simulink model "project2"  (R2023a)
settings: Solver=ode23tb  StartTime=0.0  StopTime=10.0  MaxStep=1e-3  RelTol=1e-3
InitFcn:
  | Ra=0.6;
  | La=12e-3;
  | Rf=240;
  | Lf=120;
  | j=1;
  | K=1.309;
libraries: spsDiodeLib x8, spsSeriesRLCBranchLib x6, spsMeanLib x4, slpidlib x4, spsControlledVoltageSourceLib x4, spsCurrentMeasurementLib x4, simulink x3, spsACVoltageSourceLib x2, spsDCVoltageSourceLib x2, spsVoltageMeasurementLib x2, sps_lib x1
settings Model: Creator=gaming3  LastModifiedBy=gaming3
settings SolverCC: ZeroCrossAlgorithm=Adaptive
settings DebuggingCC: IgnoredZcDiagnostic=none

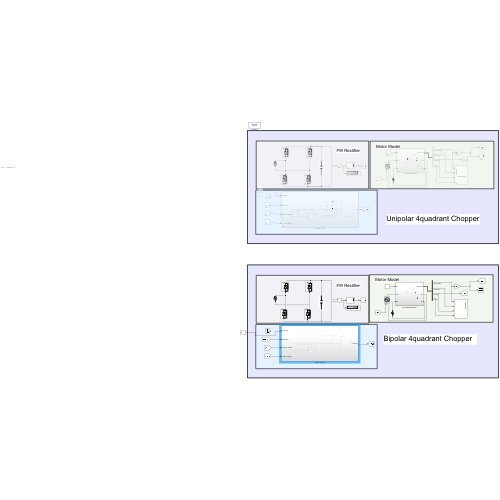
[thumbnail: Simulink's stored preview of the top-level diagram]
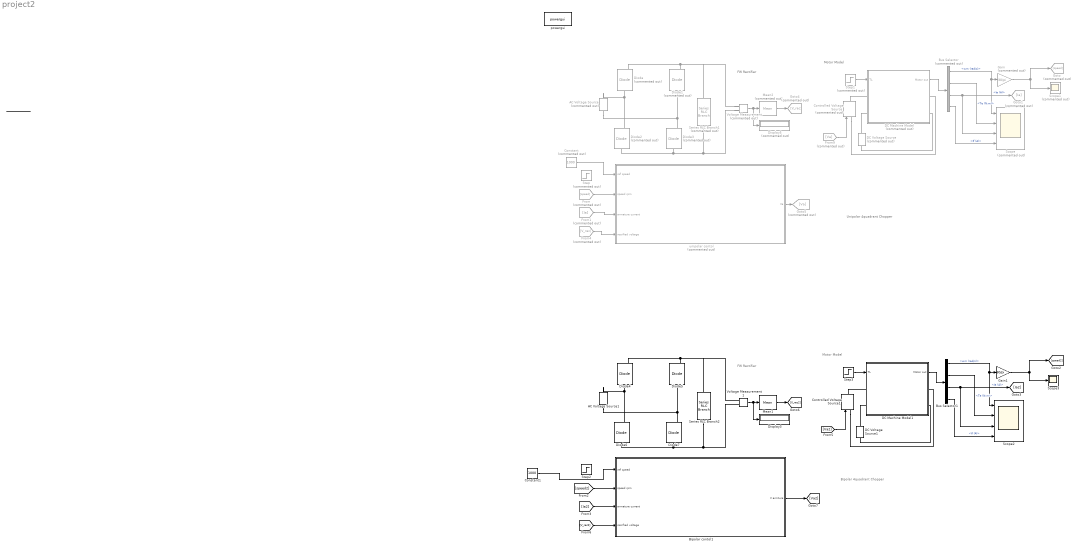
== system project2 ==
  note: Unipolar 4quadrant Chopper
  note: FW Rectifier
  note: Motor Model
  note: Bipolar 4quadrant Chopper
  note: FW Rectifier
  note: Motor Model
  AC Voltage Source : spsACVoltageSourceLib/AC Voltage Source  Commented=on  Amplitude=220  Phase=0  Frequency=50  SampleTime=0  Measurements=None  BusType=swing  Pref=10e3  Qref=0  Qmin=-inf  Qmax=+inf
  AC Voltage Source1 : spsACVoltageSourceLib/AC Voltage Source  Amplitude=220  Phase=0  Frequency=50  SampleTime=0  Measurements=None  BusType=swing  Pref=10e3  Qref=0  Qmin=-inf  Qmax=+inf
  Bipolar contol1 : Subsystem
  Bus Selector : BusSelector  Commented=on  OutputSignals=wm (rad/s),Te (N:m),Ia (A),If (A)
  Bus Selector1 : BusSelector  OutputSignals=wm (rad/s),Te (N:m),Ia (A),If (A)
  Constant : Constant  Commented=on  Value=1000
  Constant1 : Constant  Value=1000
  Controlled Voltage Source : spsControlledVoltageSourceLib/Controlled Voltage Source  Commented=on  Initialize=on  Source_Type=DC  Amplitude=0  Phase=0  Frequency=0  Measurements=None
  Controlled Voltage Source1 : spsControlledVoltageSourceLib/Controlled Voltage Source  Initialize=on  Source_Type=DC  Amplitude=0  Phase=0  Frequency=0  Measurements=None
  DC Machine Model : Subsystem  Commented=on
  DC Machine Model1 : Subsystem
  DC Voltage Source : spsDCVoltageSourceLib/DC Voltage Source  Commented=on  Amplitude=300  Measurements=None
  DC Voltage Source1 : spsDCVoltageSourceLib/DC Voltage Source  Amplitude=300  Measurements=None
  Diode{,1..3} (4 alike) : spsDiodeLib/Diode  Commented=on  Ron=0.001  Lon=0  Vf=0.8  IC=0  UseSnubber=0  Rs=500  Cs=250e-9  Measurements=on
  Diode{4..7} (4 alike) : spsDiodeLib/Diode  Ron=0.001  Lon=0  Vf=0.8  IC=0  UseSnubber=0  Rs=500  Cs=250e-9  Measurements=on
  Display3 : Display
  Display5 : Display  Commented=on
  From : From  Commented=on  GotoTag=speed
  From1 : From  Commented=on  GotoTag=Ia
  From4 : From  Commented=on  GotoTag=V_rec
  From9 : From  Commented=on  GotoTag=Va
  Gain : Gain  Commented=on  Gain=30/pi
  Gain1 : Gain  Gain=30/pi
  Goto : Goto  Commented=on  GotoTag=speed
  Goto1 : Goto  Commented=on  GotoTag=Ia
  Goto4 : Goto  Commented=on  GotoTag=V_rec
  Goto5 : Goto  Commented=on  GotoTag=Va
  Mean1 : spsMeanLib/Mean  Freq=50  Vinit=0  Ts=0
  Mean2 : spsMeanLib/Mean  Commented=on  Freq=50  Vinit=0  Ts=0
  Scope : Scope  Commented=on  NumInputPorts=4
  Scope1 : Scope  Commented=on
  Scope2 : Scope  NumInputPorts=4
  Scope3 : Scope
  Series RLC Branch1 : spsSeriesRLCBranchLib/Series RLC Branch  Commented=on  LConnTagsString=__new0  RConnTagsString=__new0  BranchType=C  Resistance=1  Inductance=1e-3  SetiL0=off  InitialCurrent=0  Capacitance=2  Setx0=off  InitialVoltage=0  Measurements=None
  Series RLC Branch2 : spsSeriesRLCBranchLib/Series RLC Branch  LConnTagsString=__new0  RConnTagsString=__new0  BranchType=C  Resistance=1  Inductance=1e-3  SetiL0=off  InitialCurrent=0  Capacitance=2  Setx0=off  InitialVoltage=0  Measurements=None
  Step : Step  Commented=on  Time=5  Before=700  After=-700  SampleTime=0
  Step1 : Step  Commented=on  Time=5  Before=70  After=100  SampleTime=0
  Step2 : Step  Time=5  Before=700  After=-700  SampleTime=0
  Step3 : Step  Time=5  Before=20  After=60  SampleTime=0
  Voltage Measurement : spsVoltageMeasurementLib/Voltage Measurement  Commented=on  PhasorSimulation=off  OutputType=Complex  PSBequivalent=0
  Voltage Measurement1 : spsVoltageMeasurementLib/Voltage Measurement  PhasorSimulation=off  OutputType=Complex  PSBequivalent=0
  powergui : sps_lib/powergui  Priority=1  SimulationMode=Discrete  SampleTime=10e-6  frequency=60  Iterations=50  frequencyindice=0  Pbase=100e6  ErrMax=1e-4  UnitsV=kV  UnitsW=MW  buscounter=0  FunctionMessages=off  echomessages=off  EnableUseOfTLC=off  CurrentSourceSwitches=off  DisableSnubberDevices=off  DisableRonSwitches=off  DisableVfSwitches=off  DisplayEquations=off  AutomaticDiscreteSolvers=off  SolverType=Tustin/Backward Euler (TBE)  Interpol=off  ExternalGateDelay=off  methode=off  Ts=100  x0status=blocks  SPID=on  SwTol=0  HookPort=off  NonlinearTolerance=1e-4  nMaxIteration=100  ContinueOnMaxIteration=off  RestoreLinks=warning  ResistiveCurrentMeasurement=off  Frange=[0:2:500]  Ylog=off  Xlog=on  ShowGrid=off  save=off  variable=ZData  structure=0  ZoomFFT=off  StartTime=0.0  cycles=1  DisplayStyle=1  fundamental=60  FreqAxis=off  MaxFrequency=1000  frequencyindicesteady=1  RmsSteady=1  display=off
  unipolar contol : Subsystem  Commented=on
  wires:
  Gain/1 -> Scope1/1, Goto/1
  Voltage Measurement/1 -> Mean2/1, Display5/1
  From/1 -> unipolar contol/2(speed rpm)
  From1/1 -> unipolar contol/3(armature current)
  Mean2/1 -> Goto4/1
  From4/1 -> unipolar contol/4(recrified voltage)
  unipolar contol/1(Va) -> Goto5/1
  Bipolar contol1/1(V armture) -> [Va2]
  [V_rec2] -> Bipolar contol1/4(recrified voltage)
  Mean1/1 -> [V_rec2]
  [Ia2] -> Bipolar contol1/3(armature current)
  [speed2] -> Bipolar contol1/2(speed rpm)
  Voltage Measurement1/1 -> Display3/1, Mean1/1
  DC Machine Model/1(Motor out) -> Bus Selector/1
  Step1/1 -> DC Machine Model/1(TL)
  From9/1 -> Controlled Voltage Source/1
  Bus Selector/1 -> Gain/1, Scope/1  "<wm (rad/s)>"
  Bus Selector/2 -> Scope/2  "<Te (N:m)>"
  Bus Selector/3 -> Goto1/1, Scope/3  "<Ia (A)>"
  Bus Selector/4 -> Scope/4  "<If (A)>"
  Bus Selector1/4 -> Scope2/4  "<If (A)>"
  Bus Selector1/3 -> Scope2/3, [Ia2]  "<Ia (A)>"
  Bus Selector1/2 -> Scope2/2  "<Te (N:m)>"
  Bus Selector1/1 -> Scope2/1, Gain1/1  "<wm (rad/s)>"
  [Va2] -> Controlled Voltage Source1/1
  Step3/1 -> DC Machine Model1/1(TL)
  DC Machine Model1/1(Motor out) -> Bus Selector1/1
  Gain1/1 -> [speed2], Scope3/1
  Constant/1 -> unipolar contol/1(ref speed)
  Constant1/1 -> Bipolar contol1/1(ref speed)
  connections:
  Diode2/RConn1 -- AC Voltage Source/RConn1 -- Diode/LConn1
  Diode3/RConn1 -- AC Voltage Source/LConn1 -- Diode1/LConn1
  Diode/RConn1 -- Voltage Measurement/LConn1 -- Series RLC Branch1/LConn1 -- Diode1/RConn1
  Series RLC Branch1/RConn1 -- Voltage Measurement/LConn2 -- Diode2/LConn1 -- Diode3/LConn1
  Diode6/RConn1 -- Diode4/LConn1 -- AC Voltage Source1/RConn1
  Diode7/RConn1 -- Diode5/LConn1 -- AC Voltage Source1/LConn1
  Diode4/RConn1 -- Diode5/RConn1 -- Series RLC Branch2/LConn1 -- Voltage Measurement1/LConn1
  Series RLC Branch2/RConn1 -- Diode7/LConn1 -- Diode6/LConn1 -- Voltage Measurement1/LConn2
  DC Voltage Source/RConn1 -- DC Machine Model/LConn2
  DC Voltage Source/LConn1 -- DC Machine Model/RConn2
  ?
  Controlled Voltage Source/RConn1 -- DC Machine Model/LConn1
  Controlled Voltage Source/LConn1 -- DC Machine Model/RConn1
  Controlled Voltage Source1/RConn1 -- DC Machine Model1/LConn1
  DC Voltage Source1/LConn1 -- DC Machine Model1/RConn2
  Controlled Voltage Source1/LConn1 -- DC Machine Model1/RConn1
  DC Voltage Source1/RConn1 -- DC Machine Model1/LConn2

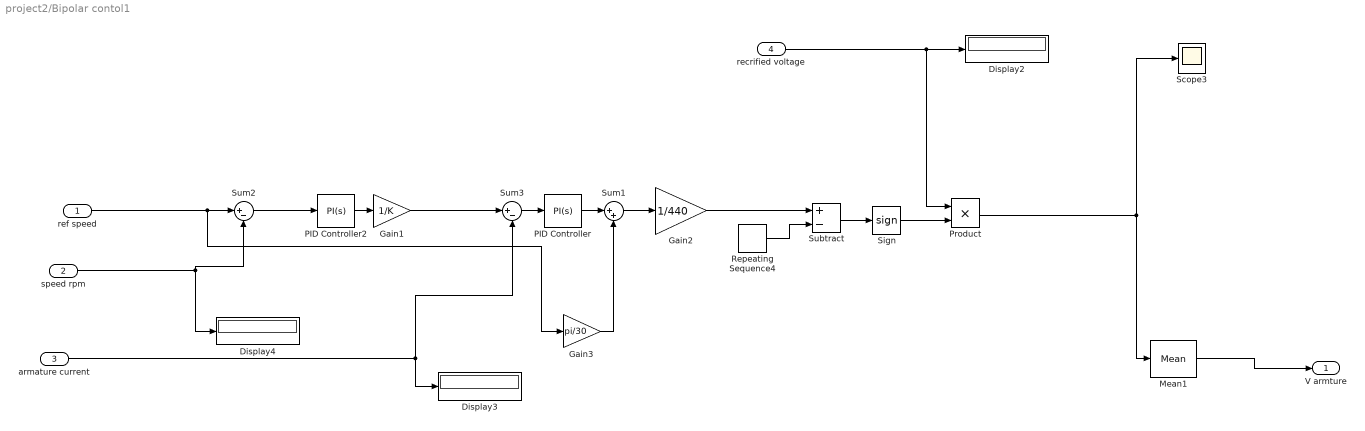
== system project2/Bipolar contol1 ==
  ref speed : Inport
  speed rpm : Inport  Port=2
  armature current : Inport  Port=3
  recrified voltage : Inport  Port=4
  Display2 : Display
  Display3 : Display
  Display4 : Display
  Gain1 : Gain  Gain=1/K
  Gain2 : Gain  Gain=1/440
  Gain3 : Gain  Gain=pi/30
  Mean1 : spsMeanLib/Mean  Freq=50  Vinit=0  Ts=0
  PID Controller : slpidlib/PID Controller  Controller=PI  Form=Parallel  TimeDomain=Continuous-time  UseExternalTs=off  SampleTime=-1  IntegratorMethod=Forward Euler  FilterMethod=Forward Euler  ControllerParametersSource=internal  P=0.01  I=10  UseKiTs=off  D=0  N=100  UseFilter=on  TunerSelectOption=Transfer Function Based (PID Tuner App)  InitialConditionSource=internal  InitialConditionForIntegrator=0  InitialConditionForFilter=0  DifferentiatorICPrevScaledInput=0  ExternalReset=none  TrackingMode=off  Kt=1  LimitOutput=on  SatLimitsSource=internal  UpperSaturationLimit=440  LowerSaturationLimit=0  LinearizeAsGain=on  AntiWindupMode=clamping  Kb=1  LimitIntegrator=off  UpperIntegratorSaturationLimit=inf  LowerIntegratorSaturationLimit=-inf  POutMin=[]  POutMax=[]  IOutMin=[]  IOutMax=[]  DOutMin=[]  DOutMax=[]  NOutMin=[]  NOutMax=[]  SumOutMin=[]  SumOutMax=[]  SaturationOutMin=[]  SaturationOutMax=[]  PParamMin=[]  PParamMax=[]  IParamMin=[]  IParamMax=[]  DParamMin=[]  DParamMax=[]  NParamMin=[]  NParamMax=[]  KbParamMin=[]  KbParamMax=[]  KtParamMin=[]  KtParamMax=[]  KbOutMin=[]  KbOutMax=[]  KtOutMin=[]  KtOutMax=[]  IntegratorOutMin=[]  IntegratorOutMax=[]  FilterOutMin=[]  FilterOutMax=[]  SumI1OutMin=[]  SumI1OutMax=[]  SumI2OutMin=[]  SumI2OutMax=[]  SumI3OutMin=[]  SumI3OutMax=[]  SumI4OutMin=[]  SumI4OutMax=[]  SumDOutMin=[]  SumDOutMax=[]  DifferentiatorOutMin=[]  DifferentiatorOutMax=[]  FilterDiffOutCoefMin=[]  FilterDiffOutCoefMax=[]  ReciprocalOutMin=[]  ReciprocalOutMax=[]  SumDenOutMin=[]  SumDenOutMax=[]  SumNumOutMin=[]  SumNumOutMax=[]  DivideOutMin=[]  DivideOutMax=[]  UdiffTsProdOutMin=[]  UdiffTsProdOutMax=[]  NTsProdOutMin=[]  NTsProdOutMax=[]  UintegralTsProdOutMin=[]  UintegralTsProdOutMax=[]  UngainTsProdOutMin=[]  UngainTsProdOutMax=[]  ClampingZeroOutDataTypeStr=Inherit: Inherit via back propagation  ClampingZeroOutMin=[]  ClampingZeroOutMax=[]  FilterDenConstantOutDataTypeStr=Inherit: Inherit via back propagation  FilterDenConstantOutMin=[]  FilterDenConstantOutMax=[]  PCopyOutDataTypeStr=Inherit: Inherit via back propagation  PCopyOutMin=[]  PCopyOutMax=[]  NCopyOutDataTypeStr=Inherit: Inherit via back propagation  NCopyOutMin=[]  NCopyOutMax=[]  IntegratorContinuousStateAttributes=''  IntegratorStateMustResolveToSignalObject=off  IntegratorRTWStateStorageClass=Auto  FilterContinuousStateAttributes=''  FilterStateMustResolveToSignalObject=off  FilterRTWStateStorageClass=Auto  ParallelPVariant=InternalParameters  IdealPVariant=Disabled  IVariant=InternalParameters  DVariant=Disabled  IntegratorVariant=Continuous  SatVariant=Enabled  AWVariant=ContClampingParallel  PCopyVariant=Disabled  TRVariant=Disabled  FdbkBlocksVariant=Forward  IdealPFdbkVariant=Disabled  SatFdbkVariant=Disabled  DerivativeFilterVariant=Disabled  NVariant=Disabled  NCopyVariant=Disabled_SignalSpec  FilterICVariant=Disabled  IntegratorICVariant=InternalICs  ExternalResetVariant=Disabled  TRSumVariant=Passthrough  SumFdbkVariant=Disabled  SumVariant=Sum_PI  TsampFilterVariant=InternalTs  TsampNgainVariant=Passthrough  TsampIntegralVariant=Disabled_SignalSpec  ExternalSaturationOutDataTypeStr=Inherit: Same as second input
  PID Controller2 : slpidlib/PID Controller  Controller=PI  Form=Parallel  TimeDomain=Continuous-time  UseExternalTs=off  SampleTime=-1  IntegratorMethod=Forward Euler  FilterMethod=Forward Euler  ControllerParametersSource=internal  P=0.5  I=0.7  UseKiTs=off  D=0  N=100  UseFilter=on  TunerSelectOption=Transfer Function Based (PID Tuner App)  InitialConditionSource=internal  InitialConditionForIntegrator=0  InitialConditionForFilter=0  DifferentiatorICPrevScaledInput=0  ExternalReset=none  TrackingMode=off  Kt=1  LimitOutput=on  SatLimitsSource=internal  UpperSaturationLimit=(30*746)/(1750*pi/30)  LowerSaturationLimit=-(30*746)/(1750*pi/30)  LinearizeAsGain=on  AntiWindupMode=clamping  Kb=1  LimitIntegrator=off  UpperIntegratorSaturationLimit=inf  LowerIntegratorSaturationLimit=-inf  POutMin=[]  POutMax=[]  IOutMin=[]  IOutMax=[]  DOutMin=[]  DOutMax=[]  NOutMin=[]  NOutMax=[]  SumOutMin=[]  SumOutMax=[]  SaturationOutMin=[]  SaturationOutMax=[]  PParamMin=[]  PParamMax=[]  IParamMin=[]  IParamMax=[]  DParamMin=[]  DParamMax=[]  NParamMin=[]  NParamMax=[]  KbParamMin=[]  KbParamMax=[]  KtParamMin=[]  KtParamMax=[]  KbOutMin=[]  KbOutMax=[]  KtOutMin=[]  KtOutMax=[]  IntegratorOutMin=[]  IntegratorOutMax=[]  FilterOutMin=[]  FilterOutMax=[]  SumI1OutMin=[]  SumI1OutMax=[]  SumI2OutMin=[]  SumI2OutMax=[]  SumI3OutMin=[]  SumI3OutMax=[]  SumI4OutMin=[]  SumI4OutMax=[]  SumDOutMin=[]  SumDOutMax=[]  DifferentiatorOutMin=[]  DifferentiatorOutMax=[]  FilterDiffOutCoefMin=[]  FilterDiffOutCoefMax=[]  ReciprocalOutMin=[]  ReciprocalOutMax=[]  SumDenOutMin=[]  SumDenOutMax=[]  SumNumOutMin=[]  SumNumOutMax=[]  DivideOutMin=[]  DivideOutMax=[]  UdiffTsProdOutMin=[]  UdiffTsProdOutMax=[]  NTsProdOutMin=[]  NTsProdOutMax=[]  UintegralTsProdOutMin=[]  UintegralTsProdOutMax=[]  UngainTsProdOutMin=[]  UngainTsProdOutMax=[]  ClampingZeroOutDataTypeStr=Inherit: Inherit via back propagation  ClampingZeroOutMin=[]  ClampingZeroOutMax=[]  FilterDenConstantOutDataTypeStr=Inherit: Inherit via back propagation  FilterDenConstantOutMin=[]  FilterDenConstantOutMax=[]  PCopyOutDataTypeStr=Inherit: Inherit via back propagation  PCopyOutMin=[]  PCopyOutMax=[]  NCopyOutDataTypeStr=Inherit: Inherit via back propagation  NCopyOutMin=[]  NCopyOutMax=[]  IntegratorContinuousStateAttributes=''  IntegratorStateMustResolveToSignalObject=off  IntegratorRTWStateStorageClass=Auto  FilterContinuousStateAttributes=''  FilterStateMustResolveToSignalObject=off  FilterRTWStateStorageClass=Auto  ParallelPVariant=InternalParameters  IdealPVariant=Disabled  IVariant=InternalParameters  DVariant=Disabled  IntegratorVariant=Continuous  SatVariant=Enabled  AWVariant=ContClampingParallel  PCopyVariant=Disabled  TRVariant=Disabled  FdbkBlocksVariant=Forward  IdealPFdbkVariant=Disabled  SatFdbkVariant=Disabled  DerivativeFilterVariant=Disabled  NVariant=Disabled  NCopyVariant=Disabled_SignalSpec  FilterICVariant=Disabled  IntegratorICVariant=InternalICs  ExternalResetVariant=Disabled  TRSumVariant=Passthrough  SumFdbkVariant=Disabled  SumVariant=Sum_PI  TsampFilterVariant=InternalTs  TsampNgainVariant=Passthrough  TsampIntegralVariant=Disabled_SignalSpec  ExternalSaturationOutDataTypeStr=Inherit: Same as second input
  Product : Product
  Repeating Sequence4 : simulink/Sources/Repeating Sequence  rep_seq_t=[0 0.5/1000 1/1000]  rep_seq_y=[0 1 0]
  Scope3 : Scope
  Sign : Signum
  Subtract : Sum  Inputs=+-
  Sum1 : Sum  Inputs=|++
  Sum2 : Sum  Inputs=|+-
  Sum3 : Sum  Inputs=|+-
  V armture : Outport
  wires:
  Sum1/1 -> Gain2/1
  Gain3/1 -> Sum1/2
  PID Controller/1 -> Sum1/1
  Gain2/1 -> Subtract/1
  Mean1/1 -> V armture/1
  Sum2/1 -> PID Controller2/1
  ref speed/1 -> Sum2/1, Gain3/1
  speed rpm/1 -> Display4/1, Sum2/2
  Gain1/1 -> Sum3/1
  armature current/1 -> Sum3/2, Display3/1
  PID Controller2/1 -> Gain1/1
  Product/1 -> Mean1/1, Scope3/1
  Sum3/1 -> PID Controller/1
  Repeating Sequence4/1 -> Subtract/2
  Subtract/1 -> Sign/1
  Sign/1 -> Product/2
  recrified voltage/1 -> Product/1, Display2/1

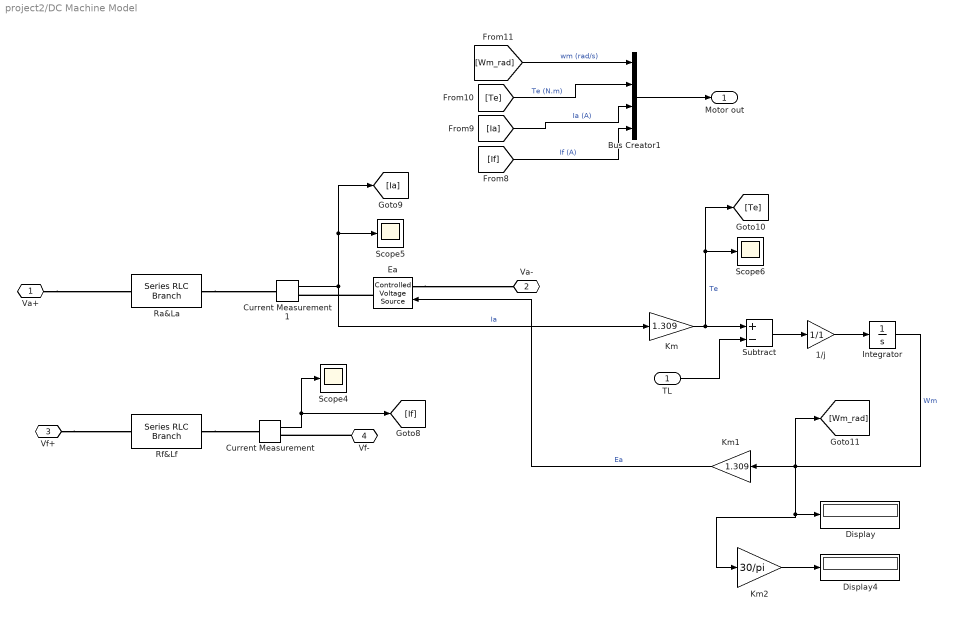
== system project2/DC Machine Model ==
  TL : Inport
  1/j : Gain  Gain=1/1
  Bus Creator1 : BusCreator  Inputs=4
  Current Measurement : spsCurrentMeasurementLib/Current Measurement  PhasorSimulation=off  OutputType=Complex  PSBequivalent=0
  Current Measurement1 : spsCurrentMeasurementLib/Current Measurement  PhasorSimulation=off  OutputType=Complex  PSBequivalent=0
  Display : Display
  Display4 : Display
  Ea : spsControlledVoltageSourceLib/Controlled Voltage Source  Initialize=on  Source_Type=AC  Amplitude=0  Phase=0  Frequency=0  Measurements=None
  Integrator : Integrator
  Km : Gain  Gain=1.309
  Km1 : Gain  Gain=1.309
  Km2 : Gain  Gain=30/pi
  Ra&La : spsSeriesRLCBranchLib/Series RLC Branch  LConnTagsString=__new0  RConnTagsString=__new0  BranchType=RL  Resistance=Ra  Inductance=La  SetiL0=off  InitialCurrent=0  Capacitance=1e-6  Setx0=off  InitialVoltage=0  Measurements=None
  Rf&Lf : spsSeriesRLCBranchLib/Series RLC Branch  LConnTagsString=__new0  RConnTagsString=__new0  BranchType=RL  Resistance=Rf  Inductance=Lf  SetiL0=off  InitialCurrent=0  Capacitance=1e-6  Setx0=off  InitialVoltage=0  Measurements=None
  Scope4 : Scope
  Scope5 : Scope
  Scope6 : Scope
  Subtract : Sum  Inputs=+-
  Va+ : PMIOPort  Side=Left
  Va- : PMIOPort  Port=2  Side=Right
  Vf+ : PMIOPort  Port=3  Side=Left
  Vf- : PMIOPort  Port=4  Side=Right
  Motor out : Outport
  wires:
  [Wm_rad] -> Bus Creator1/1  "wm (rad/s)"
  TL/1 -> Subtract/2
  Current Measurement1/1 -> Km/1, Scope5/1, [Ia]  "Ia"
  [Te] -> Bus Creator1/2  "Te (N.m)"
  Km2/1 -> Display4/1
  Bus Creator1/1 -> Motor out/1
  Current Measurement/1 -> [If], Scope4/1
  [Ia] -> Bus Creator1/3  "Ia (A)"
  Integrator/1 -> Km1/1, Display/1, Km2/1, [Wm_rad]  "Wm"
  Km/1 -> Subtract/1, Scope6/1, [Te]  "Te"
  Subtract/1 -> 1/j/1
  Km1/1 -> Ea/1  "Ea"
  [If] -> Bus Creator1/4  "If (A)"
  1/j/1 -> Integrator/1
  connections:
  Vf+/RConn1 -- Rf&Lf/LConn1
  Ea/RConn1 -- Current Measurement1/RConn1
  Vf-/RConn1 -- Current Measurement/RConn1
  Ra&La/RConn1 -- Current Measurement1/LConn1
  Rf&Lf/RConn1 -- Current Measurement/LConn1
  Ea/LConn1 -- Va-/RConn1
  Va+/RConn1 -- Ra&La/LConn1

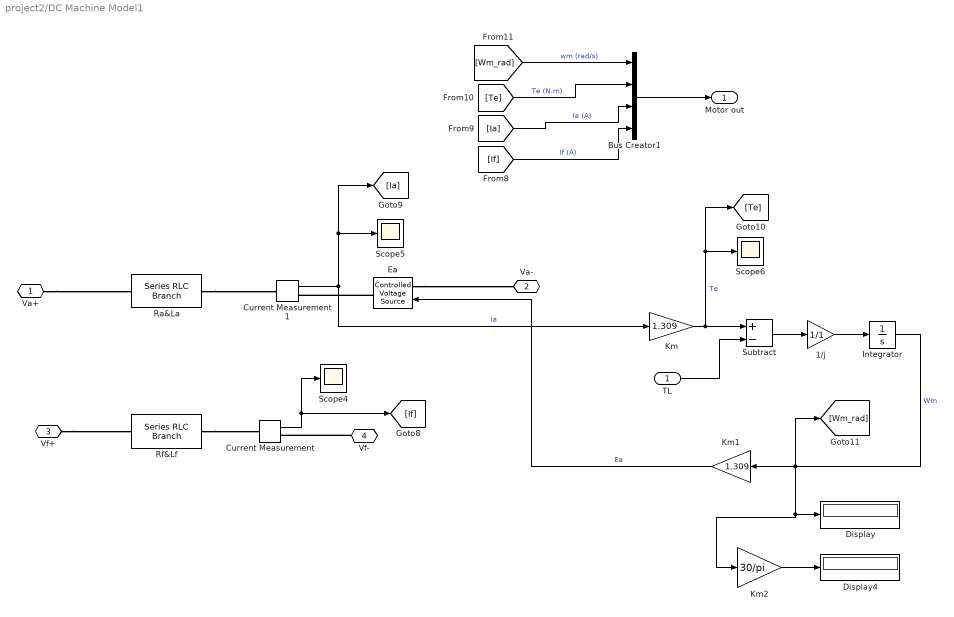
== system project2/DC Machine Model1 ==
  TL : Inport
  1/j : Gain  Gain=1/1
  Bus Creator1 : BusCreator  Inputs=4
  Current Measurement : spsCurrentMeasurementLib/Current Measurement  PhasorSimulation=off  OutputType=Complex  PSBequivalent=0
  Current Measurement1 : spsCurrentMeasurementLib/Current Measurement  PhasorSimulation=off  OutputType=Complex  PSBequivalent=0
  Display : Display
  Display4 : Display
  Ea : spsControlledVoltageSourceLib/Controlled Voltage Source  Initialize=on  Source_Type=AC  Amplitude=0  Phase=0  Frequency=0  Measurements=None
  Integrator : Integrator
  Km : Gain  Gain=1.309
  Km1 : Gain  Gain=1.309
  Km2 : Gain  Gain=30/pi
  Ra&La : spsSeriesRLCBranchLib/Series RLC Branch  LConnTagsString=__new0  RConnTagsString=__new0  BranchType=RL  Resistance=Ra  Inductance=La  SetiL0=off  InitialCurrent=0  Capacitance=1e-6  Setx0=off  InitialVoltage=0  Measurements=None
  Rf&Lf : spsSeriesRLCBranchLib/Series RLC Branch  LConnTagsString=__new0  RConnTagsString=__new0  BranchType=RL  Resistance=Rf  Inductance=Lf  SetiL0=off  InitialCurrent=0  Capacitance=1e-6  Setx0=off  InitialVoltage=0  Measurements=None
  Scope4 : Scope
  Scope5 : Scope
  Scope6 : Scope
  Subtract : Sum  Inputs=+-
  Va+ : PMIOPort  Side=Left
  Va- : PMIOPort  Port=2  Side=Right
  Vf+ : PMIOPort  Port=3  Side=Left
  Vf- : PMIOPort  Port=4  Side=Right
  Motor out : Outport
  wires:
  1/j/1 -> Integrator/1
  [If] -> Bus Creator1/4  "If (A)"
  Km1/1 -> Ea/1  "Ea"
  Subtract/1 -> 1/j/1
  Km/1 -> [Te], Scope6/1, Subtract/1  "Te"
  Integrator/1 -> [Wm_rad], Km2/1, Display/1, Km1/1  "Wm"
  [Ia] -> Bus Creator1/3  "Ia (A)"
  Current Measurement/1 -> Scope4/1, [If]
  Bus Creator1/1 -> Motor out/1
  Km2/1 -> Display4/1
  [Te] -> Bus Creator1/2  "Te (N.m)"
  Current Measurement1/1 -> [Ia], Scope5/1, Km/1  "Ia"
  TL/1 -> Subtract/2
  [Wm_rad] -> Bus Creator1/1  "wm (rad/s)"
  connections:
  Va+/RConn1 -- Ra&La/LConn1
  Ea/LConn1 -- Va-/RConn1
  Rf&Lf/RConn1 -- Current Measurement/LConn1
  Ra&La/RConn1 -- Current Measurement1/LConn1
  Vf-/RConn1 -- Current Measurement/RConn1
  Ea/RConn1 -- Current Measurement1/RConn1
  Vf+/RConn1 -- Rf&Lf/LConn1

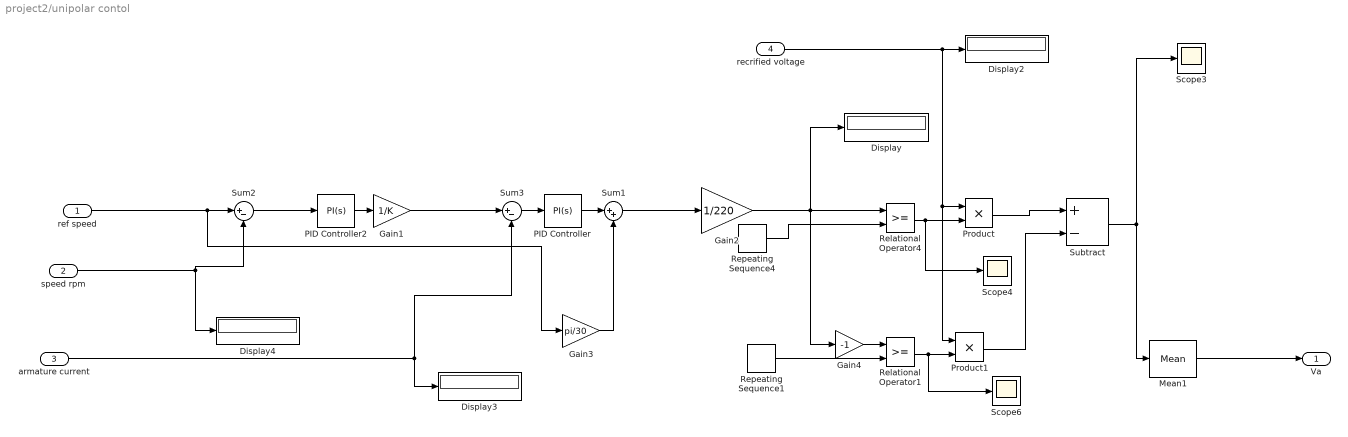
== system project2/unipolar contol ==
  ref speed : Inport
  speed rpm : Inport  Port=2
  armature current : Inport  Port=3
  recrified voltage : Inport  Port=4
  Display{,2..4} (4 alike) : Display
  Gain1 : Gain  Gain=1/K
  Gain2 : Gain  Gain=1/220
  Gain3 : Gain  Gain=pi/30
  Gain4 : Gain  Gain=-1
  Mean1 : spsMeanLib/Mean  Freq=50  Vinit=0  Ts=0
  PID Controller : slpidlib/PID Controller  Controller=PI  Form=Parallel  TimeDomain=Continuous-time  UseExternalTs=off  SampleTime=-1  IntegratorMethod=Forward Euler  FilterMethod=Forward Euler  ControllerParametersSource=internal  P=0.1  I=1  UseKiTs=off  D=0  N=100  UseFilter=on  TunerSelectOption=Transfer Function Based (PID Tuner App)  InitialConditionSource=internal  InitialConditionForIntegrator=0  InitialConditionForFilter=0  DifferentiatorICPrevScaledInput=0  ExternalReset=none  TrackingMode=off  Kt=1  LimitOutput=on  SatLimitsSource=internal  UpperSaturationLimit=220  LowerSaturationLimit=-220  LinearizeAsGain=on  AntiWindupMode=clamping  Kb=1  LimitIntegrator=off  UpperIntegratorSaturationLimit=inf  LowerIntegratorSaturationLimit=-inf  POutMin=[]  POutMax=[]  IOutMin=[]  IOutMax=[]  DOutMin=[]  DOutMax=[]  NOutMin=[]  NOutMax=[]  SumOutMin=[]  SumOutMax=[]  SaturationOutMin=[]  SaturationOutMax=[]  PParamMin=[]  PParamMax=[]  IParamMin=[]  IParamMax=[]  DParamMin=[]  DParamMax=[]  NParamMin=[]  NParamMax=[]  KbParamMin=[]  KbParamMax=[]  KtParamMin=[]  KtParamMax=[]  KbOutMin=[]  KbOutMax=[]  KtOutMin=[]  KtOutMax=[]  IntegratorOutMin=[]  IntegratorOutMax=[]  FilterOutMin=[]  FilterOutMax=[]  SumI1OutMin=[]  SumI1OutMax=[]  SumI2OutMin=[]  SumI2OutMax=[]  SumI3OutMin=[]  SumI3OutMax=[]  SumI4OutMin=[]  SumI4OutMax=[]  SumDOutMin=[]  SumDOutMax=[]  DifferentiatorOutMin=[]  DifferentiatorOutMax=[]  FilterDiffOutCoefMin=[]  FilterDiffOutCoefMax=[]  ReciprocalOutMin=[]  ReciprocalOutMax=[]  SumDenOutMin=[]  SumDenOutMax=[]  SumNumOutMin=[]  SumNumOutMax=[]  DivideOutMin=[]  DivideOutMax=[]  UdiffTsProdOutMin=[]  UdiffTsProdOutMax=[]  NTsProdOutMin=[]  NTsProdOutMax=[]  UintegralTsProdOutMin=[]  UintegralTsProdOutMax=[]  UngainTsProdOutMin=[]  UngainTsProdOutMax=[]  ClampingZeroOutDataTypeStr=Inherit: Inherit via back propagation  ClampingZeroOutMin=[]  ClampingZeroOutMax=[]  FilterDenConstantOutDataTypeStr=Inherit: Inherit via back propagation  FilterDenConstantOutMin=[]  FilterDenConstantOutMax=[]  PCopyOutDataTypeStr=Inherit: Inherit via back propagation  PCopyOutMin=[]  PCopyOutMax=[]  NCopyOutDataTypeStr=Inherit: Inherit via back propagation  NCopyOutMin=[]  NCopyOutMax=[]  IntegratorContinuousStateAttributes=''  IntegratorStateMustResolveToSignalObject=off  IntegratorRTWStateStorageClass=Auto  FilterContinuousStateAttributes=''  FilterStateMustResolveToSignalObject=off  FilterRTWStateStorageClass=Auto  ParallelPVariant=InternalParameters  IdealPVariant=Disabled  IVariant=InternalParameters  DVariant=Disabled  IntegratorVariant=Continuous  SatVariant=Enabled  AWVariant=ContClampingParallel  PCopyVariant=Disabled  TRVariant=Disabled  FdbkBlocksVariant=Forward  IdealPFdbkVariant=Disabled  SatFdbkVariant=Disabled  DerivativeFilterVariant=Disabled  NVariant=Disabled  NCopyVariant=Disabled_SignalSpec  FilterICVariant=Disabled  IntegratorICVariant=InternalICs  ExternalResetVariant=Disabled  TRSumVariant=Passthrough  SumFdbkVariant=Disabled  SumVariant=Sum_PI  TsampFilterVariant=InternalTs  TsampNgainVariant=Passthrough  TsampIntegralVariant=Disabled_SignalSpec  ExternalSaturationOutDataTypeStr=Inherit: Same as second input
  PID Controller2 : slpidlib/PID Controller  Controller=PI  Form=Parallel  TimeDomain=Continuous-time  UseExternalTs=off  SampleTime=-1  IntegratorMethod=Forward Euler  FilterMethod=Forward Euler  ControllerParametersSource=internal  P=0.5  I=0.5  UseKiTs=off  D=0  N=100  UseFilter=on  TunerSelectOption=Transfer Function Based (PID Tuner App)  InitialConditionSource=internal  InitialConditionForIntegrator=0  InitialConditionForFilter=0  DifferentiatorICPrevScaledInput=0  ExternalReset=none  TrackingMode=off  Kt=1  LimitOutput=on  SatLimitsSource=internal  UpperSaturationLimit=(30*746)/(1750*pi/30)  LowerSaturationLimit=-(30*746)/(1750*pi/30)  LinearizeAsGain=on  AntiWindupMode=clamping  Kb=1  LimitIntegrator=off  UpperIntegratorSaturationLimit=inf  LowerIntegratorSaturationLimit=-inf  POutMin=[]  POutMax=[]  IOutMin=[]  IOutMax=[]  DOutMin=[]  DOutMax=[]  NOutMin=[]  NOutMax=[]  SumOutMin=[]  SumOutMax=[]  SaturationOutMin=[]  SaturationOutMax=[]  PParamMin=[]  PParamMax=[]  IParamMin=[]  IParamMax=[]  DParamMin=[]  DParamMax=[]  NParamMin=[]  NParamMax=[]  KbParamMin=[]  KbParamMax=[]  KtParamMin=[]  KtParamMax=[]  KbOutMin=[]  KbOutMax=[]  KtOutMin=[]  KtOutMax=[]  IntegratorOutMin=[]  IntegratorOutMax=[]  FilterOutMin=[]  FilterOutMax=[]  SumI1OutMin=[]  SumI1OutMax=[]  SumI2OutMin=[]  SumI2OutMax=[]  SumI3OutMin=[]  SumI3OutMax=[]  SumI4OutMin=[]  SumI4OutMax=[]  SumDOutMin=[]  SumDOutMax=[]  DifferentiatorOutMin=[]  DifferentiatorOutMax=[]  FilterDiffOutCoefMin=[]  FilterDiffOutCoefMax=[]  ReciprocalOutMin=[]  ReciprocalOutMax=[]  SumDenOutMin=[]  SumDenOutMax=[]  SumNumOutMin=[]  SumNumOutMax=[]  DivideOutMin=[]  DivideOutMax=[]  UdiffTsProdOutMin=[]  UdiffTsProdOutMax=[]  NTsProdOutMin=[]  NTsProdOutMax=[]  UintegralTsProdOutMin=[]  UintegralTsProdOutMax=[]  UngainTsProdOutMin=[]  UngainTsProdOutMax=[]  ClampingZeroOutDataTypeStr=Inherit: Inherit via back propagation  ClampingZeroOutMin=[]  ClampingZeroOutMax=[]  FilterDenConstantOutDataTypeStr=Inherit: Inherit via back propagation  FilterDenConstantOutMin=[]  FilterDenConstantOutMax=[]  PCopyOutDataTypeStr=Inherit: Inherit via back propagation  PCopyOutMin=[]  PCopyOutMax=[]  NCopyOutDataTypeStr=Inherit: Inherit via back propagation  NCopyOutMin=[]  NCopyOutMax=[]  IntegratorContinuousStateAttributes=''  IntegratorStateMustResolveToSignalObject=off  IntegratorRTWStateStorageClass=Auto  FilterContinuousStateAttributes=''  FilterStateMustResolveToSignalObject=off  FilterRTWStateStorageClass=Auto  ParallelPVariant=InternalParameters  IdealPVariant=Disabled  IVariant=InternalParameters  DVariant=Disabled  IntegratorVariant=Continuous  SatVariant=Enabled  AWVariant=ContClampingParallel  PCopyVariant=Disabled  TRVariant=Disabled  FdbkBlocksVariant=Forward  IdealPFdbkVariant=Disabled  SatFdbkVariant=Disabled  DerivativeFilterVariant=Disabled  NVariant=Disabled  NCopyVariant=Disabled_SignalSpec  FilterICVariant=Disabled  IntegratorICVariant=InternalICs  ExternalResetVariant=Disabled  TRSumVariant=Passthrough  SumFdbkVariant=Disabled  SumVariant=Sum_PI  TsampFilterVariant=InternalTs  TsampNgainVariant=Passthrough  TsampIntegralVariant=Disabled_SignalSpec  ExternalSaturationOutDataTypeStr=Inherit: Same as second input
  Product : Product
  Product1 : Product
  Relational Operator1 : RelationalOperator  OutDataTypeStr=boolean  RndMeth=Simplest  InputSameDT=off
  Relational Operator4 : RelationalOperator  OutDataTypeStr=boolean  RndMeth=Simplest  InputSameDT=off
  Repeating Sequence1 : simulink/Sources/Repeating Sequence  rep_seq_t=[0 0.5/1000 1/1000]  rep_seq_y=[-1 0 -1]
  Repeating Sequence4 : simulink/Sources/Repeating Sequence  rep_seq_t=[0 0.5/1000 1/1000]  rep_seq_y=[0 1 0]
  Scope3 : Scope
  Scope4 : Scope
  Scope6 : Scope
  Subtract : Sum  Inputs=+-
  Sum1 : Sum  Inputs=|++
  Sum2 : Sum  Inputs=|+-
  Sum3 : Sum  Inputs=|+-
  Va : Outport
  wires:
  Sum3/1 -> PID Controller/1
  Relational Operator1/1 -> Scope6/1, Product1/2
  Subtract/1 -> Scope3/1, Mean1/1
  Repeating Sequence1/1 -> Relational Operator1/2
  PID Controller2/1 -> Gain1/1
  Relational Operator4/1 -> Scope4/1, Product/2
  Product/1 -> Subtract/1
  armature current/1 -> Display3/1, Sum3/2
  Product1/1 -> Subtract/2
  Gain4/1 -> Relational Operator1/1
  Gain1/1 -> Sum3/1
  speed rpm/1 -> Sum2/2, Display4/1
  Repeating Sequence4/1 -> Relational Operator4/2
  ref speed/1 -> Gain3/1, Sum2/1
  Sum2/1 -> PID Controller2/1
  Mean1/1 -> Va/1
  Gain2/1 -> Gain4/1, Relational Operator4/1, Display/1
  recrified voltage/1 -> Product1/1, Product/1, Display2/1
  PID Controller/1 -> Sum1/1
  Gain3/1 -> Sum1/2
  Sum1/1 -> Gain2/1
  ? -> ?
